simulink subsystem "Joystick_Input_To_Swerve_Drive_sub"  (R2023b)
settings: Solver=VariableStepAuto  StartTime=0.0  StopTime=10.0  RelTol=1e-3
undefined symbols (not defined in the file): Boost_Trigger_High_Speed, Boost_Trigger_Low_Speed, Steering_Abs_Deadband_Range, Steering_Mod_Drv_in, Steering_Mod_Drv_out, Steering_Mod_Str_Rel_in, Steering_Mod_Str_Rel_out, Steering_Relative_Gain
libraries: hdlsllib x5, simulink x4, simulink_extras x1, Controls_Components_lib x1
settings Model: Creator=ander  LastModifiedBy=FIRSTMentor

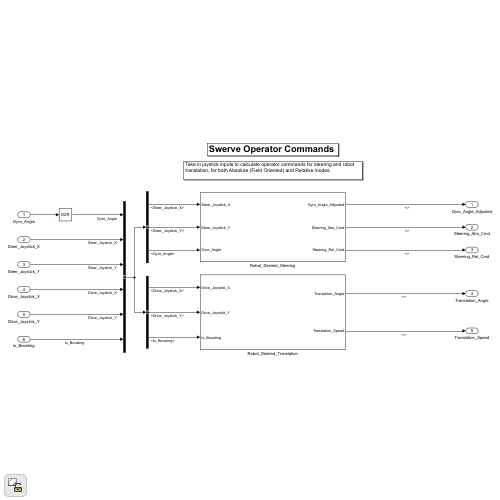
[thumbnail: Simulink's stored preview of the top-level diagram]
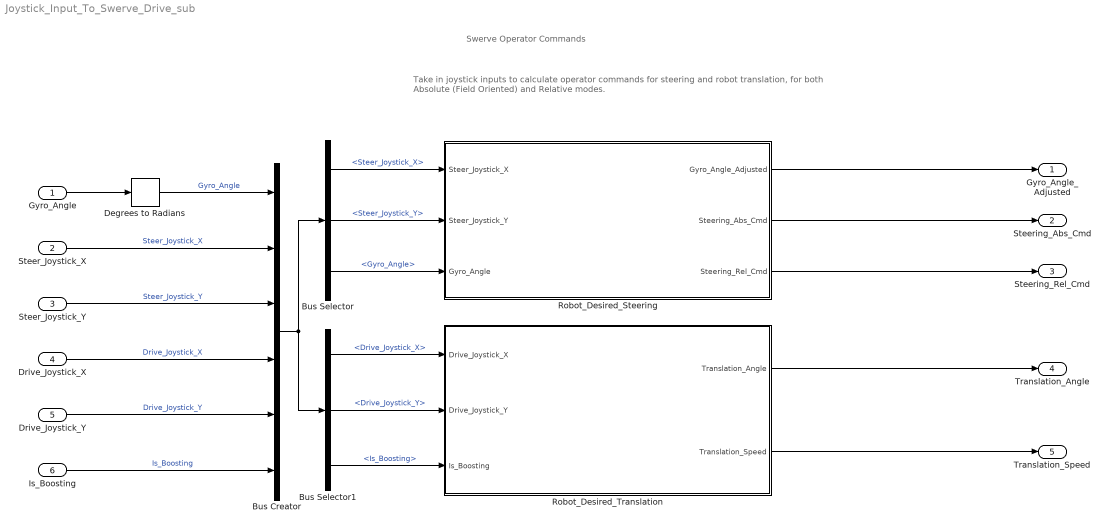
== system Joystick_Input_To_Swerve_Drive_sub ==
  note: Take in joystick inputs to calculate operator commands for steering and robot translation, for both Absolute (Field Oriented) and Relative modes.
  note: Swerve Operator Commands
  Gyro_Angle : Inport
  Steer_Joystick_X : Inport  Port=2
  Steer_Joystick_Y : Inport  Port=3
  Drive_Joystick_X : Inport  Port=4
  Drive_Joystick_Y : Inport  Port=5
  Is_Boosting : Inport  Port=6
  Bus Creator : BusCreator  Inputs=6
  Bus Selector : BusSelector  OutputSignals=Steer_Joystick_X,Steer_Joystick_Y,Gyro_Angle
  Bus Selector1 : BusSelector  OutputSignals=Drive_Joystick_X,Drive_Joystick_Y,Is_Boosting
  Degrees to Radians : simulink_extras/Transformations/Degrees to Radians
  Robot_Desired_Steering : Subsystem
  Robot_Desired_Translation : Subsystem
  Gyro_Angle_Adjusted : Outport
  Steering_Abs_Cmd : Outport  Port=2
  Steering_Rel_Cmd : Outport  Port=3
  Translation_Angle : Outport  Port=4
  Translation_Speed : Outport  Port=5
  wires:
  Drive_Joystick_X/1 -> Bus Creator/4  "Drive_Joystick_X"
  Drive_Joystick_Y/1 -> Bus Creator/5  "Drive_Joystick_Y"
  Steer_Joystick_X/1 -> Bus Creator/2  "Steer_Joystick_X"
  Bus Selector1/1 -> Robot_Desired_Translation/1(Drive_Joystick_X)  "<Drive_Joystick_X>"
  Bus Selector1/2 -> Robot_Desired_Translation/2(Drive_Joystick_Y)  "<Drive_Joystick_Y>"
  Steer_Joystick_Y/1 -> Bus Creator/3  "Steer_Joystick_Y"
  Degrees to Radians/1 -> Bus Creator/1  "Gyro_Angle"
  Gyro_Angle/1 -> Degrees to Radians/1
  Bus Creator/1 -> Bus Selector/1, Bus Selector1/1
  Robot_Desired_Translation/2(Translation_Speed) -> Translation_Speed/1
  Robot_Desired_Translation/1(Translation_Angle) -> Translation_Angle/1
  Bus Selector/1 -> Robot_Desired_Steering/1(Steer_Joystick_X)  "<Steer_Joystick_X>"
  Bus Selector/2 -> Robot_Desired_Steering/2(Steer_Joystick_Y)  "<Steer_Joystick_Y>"
  Bus Selector/3 -> Robot_Desired_Steering/3(Gyro_Angle)  "<Gyro_Angle>"
  Robot_Desired_Steering/1(Gyro_Angle_Adjusted) -> Gyro_Angle_Adjusted/1
  Robot_Desired_Steering/2(Steering_Abs_Cmd) -> Steering_Abs_Cmd/1
  Robot_Desired_Steering/3(Steering_Rel_Cmd) -> Steering_Rel_Cmd/1
  Is_Boosting/1 -> Bus Creator/6  "Is_Boosting"
  Bus Selector1/3 -> Robot_Desired_Translation/3(Is_Boosting)  "<Is_Boosting>"

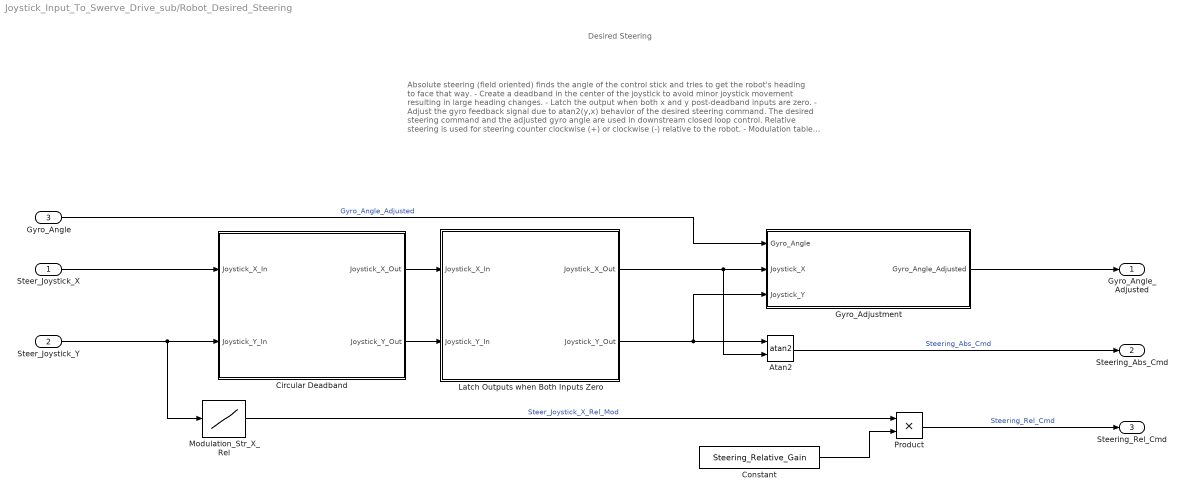
== system Joystick_Input_To_Swerve_Drive_sub/Robot_Desired_Steering ==
  note: Absolute steering (field oriented) finds the angle of the control stick and tries to get the robot's heading to face that way.
      | - Create a deadband in the center of the joystick to avoid minor joystick movement resulting in large heading changes.
      | - Latch the output when both x and y post-deadband inputs are zero.
      | - Adjust the gyro feedback signal due to atan2(y,x) behavior of the desired steering command. The desired steering command and the adjusted gyro angle are used in downstream closed loop control.
      |
      | Relative steering is used for steering counter clockwise (+) or clockwise (-) relative to the robot.
      | - Modulation table for joystick input. Only one axis of the steering joystck is used.
      | - The gain block adjusts how fast the robot will rotate.
  note: Desired Steering
  Steer_Joystick_X : Inport
  Steer_Joystick_Y : Inport  Port=2
  Gyro_Angle : Inport  Port=3
  Atan2 : Trigonometry  Operator=atan2
  Circular Deadband : Subsystem
  Constant : Constant  Value=Steering_Relative_Gain
  Gyro_Adjustment : Subsystem
  Latch Outputs when Both Inputs Zero : Subsystem
  Modulation_Str_X_Rel : Lookup_n-D  NumberOfTableDimensions=1  BreakpointsForDimension1=Steering_Mod_Str_Rel_in  Table=Steering_Mod_Str_Rel_out  ExtrapMethod=Clip  InternalRulePriority=Speed  RndMeth=Simplest
  Product : Product
  Gyro_Angle_Adjusted : Outport
  Steering_Abs_Cmd : Outport  Port=2
  Steering_Rel_Cmd : Outport  Port=3
  wires:
  Latch Outputs when Both Inputs Zero/1(Joystick_X_Out) -> Gyro_Adjustment/2(Joystick_X), Atan2/2
  Circular Deadband/1(Joystick_X_Out) -> Latch Outputs when Both Inputs Zero/1(Joystick_X_In)
  Circular Deadband/2(Joystick_Y_Out) -> Latch Outputs when Both Inputs Zero/2(Joystick_Y_In)
  Steer_Joystick_Y/1 -> Circular Deadband/2(Joystick_Y_In), Modulation_Str_X_Rel/1
  Latch Outputs when Both Inputs Zero/2(Joystick_Y_Out) -> Atan2/1, Gyro_Adjustment/3(Joystick_Y)
  Gyro_Adjustment/1(Gyro_Angle_Adjusted) -> Gyro_Angle_Adjusted/1
  Gyro_Angle/1 -> Gyro_Adjustment/1(Gyro_Angle)  "Gyro_Angle_Adjusted"
  Atan2/1 -> Steering_Abs_Cmd/1  "Steering_Abs_Cmd"
  Constant/1 -> Product/2
  Product/1 -> Steering_Rel_Cmd/1  "Steering_Rel_Cmd"
  Steer_Joystick_X/1 -> Circular Deadband/1(Joystick_X_In)
  Modulation_Str_X_Rel/1 -> Product/1  "Steer_Joystick_X_Rel_Mod"

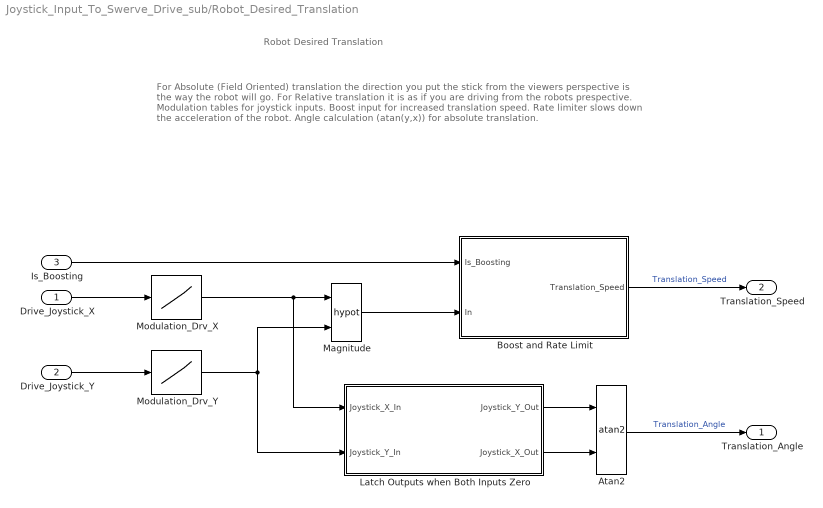
== system Joystick_Input_To_Swerve_Drive_sub/Robot_Desired_Translation ==
  note: Robot Desired Translation
  note: For Absolute (Field Oriented) translation the direction you put the stick from the viewers perspective is the way the robot will go.
      |
      | For Relative translation it is as if you are driving from the robots prespective.
      |
      | Modulation tables for joystick inputs.
      | Boost input for increased translation speed.
      | Rate limiter slows down the acceleration of the robot.
      | Angle calculation (atan(y,x)) for absolute translation.
  Drive_Joystick_X : Inport
  Drive_Joystick_Y : Inport  Port=2
  Is_Boosting : Inport  Port=3
  Atan2 : Trigonometry  Operator=atan2
  Boost and Rate Limit : Subsystem
  Latch Outputs when Both Inputs Zero : Subsystem
  Magnitude : Math  Operator=hypot
  Modulation_Drv_X : Lookup_n-D  NumberOfTableDimensions=1  BreakpointsForDimension1=Steering_Mod_Drv_in  Table=Steering_Mod_Drv_out  ExtrapMethod=Clip  InternalRulePriority=Speed  RndMeth=Simplest
  Modulation_Drv_Y : Lookup_n-D  NumberOfTableDimensions=1  BreakpointsForDimension1=Steering_Mod_Drv_in  Table=Steering_Mod_Drv_out  ExtrapMethod=Clip  InternalRulePriority=Speed  RndMeth=Simplest
  Translation_Angle : Outport
  Translation_Speed : Outport  Port=2
  wires:
  Modulation_Drv_Y/1 -> Magnitude/2, Latch Outputs when Both Inputs Zero/2(Joystick_Y_In)
  Latch Outputs when Both Inputs Zero/1(Joystick_Y_Out) -> Atan2/1
  Latch Outputs when Both Inputs Zero/2(Joystick_X_Out) -> Atan2/2
  Is_Boosting/1 -> Boost and Rate Limit/1(Is_Boosting)
  Boost and Rate Limit/1(Translation_Speed) -> Translation_Speed/1  "Translation_Speed"
  Modulation_Drv_X/1 -> Magnitude/1, Latch Outputs when Both Inputs Zero/1(Joystick_X_In)
  Atan2/1 -> Translation_Angle/1  "Translation_Angle"
  Magnitude/1 -> Boost and Rate Limit/2(In)
  Drive_Joystick_X/1 -> Modulation_Drv_X/1
  Drive_Joystick_Y/1 -> Modulation_Drv_Y/1

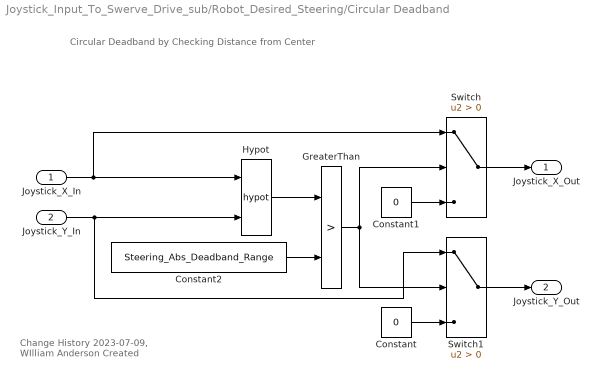
== system Joystick_Input_To_Swerve_Drive_sub/Robot_Desired_Steering/Circular Deadband ==
  note: Circular Deadband by Checking Distance from Center
  note: Change History
      | 2023-07-09, WIlliam Anderson
      | Created
  Joystick_X_In : Inport
  Joystick_Y_In : Inport  Port=2
  Constant : Constant  Value=0
  Constant1 : Constant  Value=0
  Constant2 : Constant  Value=Steering_Abs_Deadband_Range
  GreaterThan : RelationalOperator  Operator=>  OutDataTypeStr=boolean  RndMeth=Simplest  InputSameDT=off
  Hypot : Math  Operator=hypot
  Switch : Switch  Criteria=u2 > Threshold  SaturateOnIntegerOverflow=off  InputSameDT=off
  Switch1 : Switch  Criteria=u2 > Threshold  SaturateOnIntegerOverflow=off  InputSameDT=off
  Joystick_X_Out : Outport
  Joystick_Y_Out : Outport  Port=2
  wires:
  GreaterThan/1 -> Switch1/2, Switch/2
  Constant2/1 -> GreaterThan/2
  Hypot/1 -> GreaterThan/1
  Joystick_Y_In/1 -> Hypot/2, Switch1/1
  Joystick_X_In/1 -> Switch/1, Hypot/1
  Constant1/1 -> Switch/3
  Constant/1 -> Switch1/3
  Switch/1 -> Joystick_X_Out/1
  Switch1/1 -> Joystick_Y_Out/1

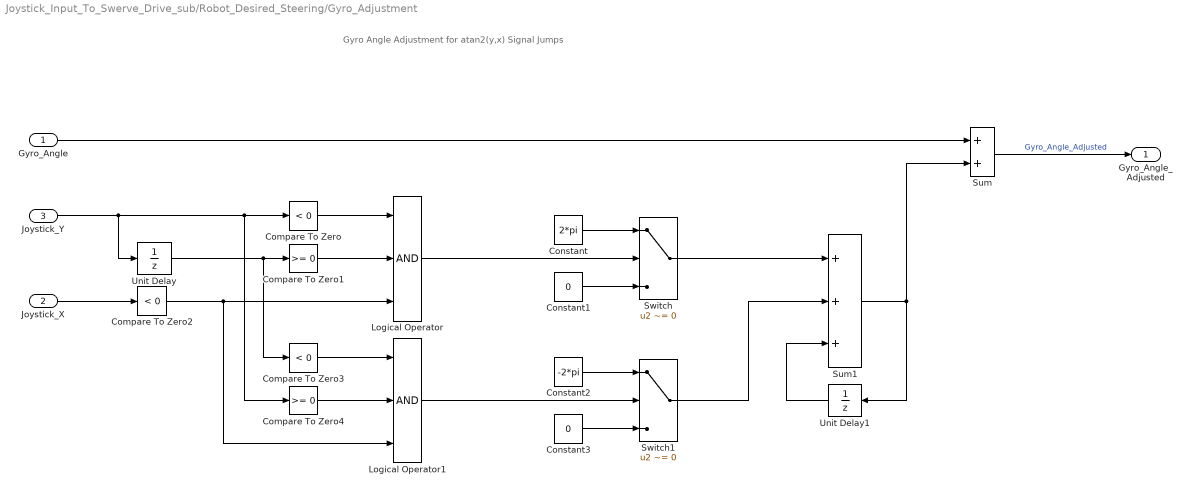
== system Joystick_Input_To_Swerve_Drive_sub/Robot_Desired_Steering/Gyro_Adjustment ==
  note: Gyro Angle Adjustment for atan2(y,x) Signal Jumps
  Gyro_Angle : Inport
  Joystick_X : Inport  Port=2
  Joystick_Y : Inport  Port=3
  Compare To Zero : hdlsllib/Logic and Bit Operations/Compare To Zero  relop=<  OutDataTypeStr=boolean
  Compare To Zero1 : hdlsllib/Logic and Bit Operations/Compare To Zero  relop=>=  OutDataTypeStr=boolean
  Compare To Zero2 : hdlsllib/Logic and Bit Operations/Compare To Zero  relop=<  OutDataTypeStr=boolean
  Compare To Zero3 : hdlsllib/Logic and Bit Operations/Compare To Zero  relop=<  OutDataTypeStr=boolean
  Compare To Zero4 : hdlsllib/Logic and Bit Operations/Compare To Zero  relop=>=  OutDataTypeStr=boolean
  Constant : Constant  Value=2*pi
  Constant1 : Constant  Value=0
  Constant2 : Constant  Value=-2*pi
  Constant3 : Constant  Value=0
  Logical Operator : Logic  Inputs=3  AllPortsSameDT=off  OutDataTypeStr=boolean
  Logical Operator1 : Logic  Inputs=3  AllPortsSameDT=off  OutDataTypeStr=boolean
  Sum : Sum  Inputs=2
  Sum1 : Sum  Inputs=3
  Switch : Switch  Criteria=u2 ~= 0  SaturateOnIntegerOverflow=off  InputSameDT=off
  Switch1 : Switch  Criteria=u2 ~= 0  SaturateOnIntegerOverflow=off  InputSameDT=off
  Unit Delay : UnitDelay  SampleTime=-1  HasFrameUpgradeWarning=on
  Unit Delay1 : UnitDelay  SampleTime=-1  HasFrameUpgradeWarning=on
  Gyro_Angle_Adjusted : Outport
  wires:
  Joystick_Y/1 -> Compare To Zero4/1, Compare To Zero/1, Unit Delay/1
  Unit Delay/1 -> Compare To Zero3/1, Compare To Zero1/1
  Compare To Zero/1 -> Logical Operator/1
  Compare To Zero1/1 -> Logical Operator/2
  Constant/1 -> Switch/1
  Constant1/1 -> Switch/3
  Logical Operator/1 -> Switch/2
  Gyro_Angle/1 -> Sum/1
  Sum/1 -> Gyro_Angle_Adjusted/1  "Gyro_Angle_Adjusted"
  Sum1/1 -> Sum/2, Unit Delay1/1
  Switch/1 -> Sum1/1
  Unit Delay1/1 -> Sum1/3
  Joystick_X/1 -> Compare To Zero2/1
  Compare To Zero2/1 -> Logical Operator1/3, Logical Operator/3
  Compare To Zero3/1 -> Logical Operator1/1
  Compare To Zero4/1 -> Logical Operator1/2
  Logical Operator1/1 -> Switch1/2
  Constant3/1 -> Switch1/3
  Constant2/1 -> Switch1/1
  Switch1/1 -> Sum1/2

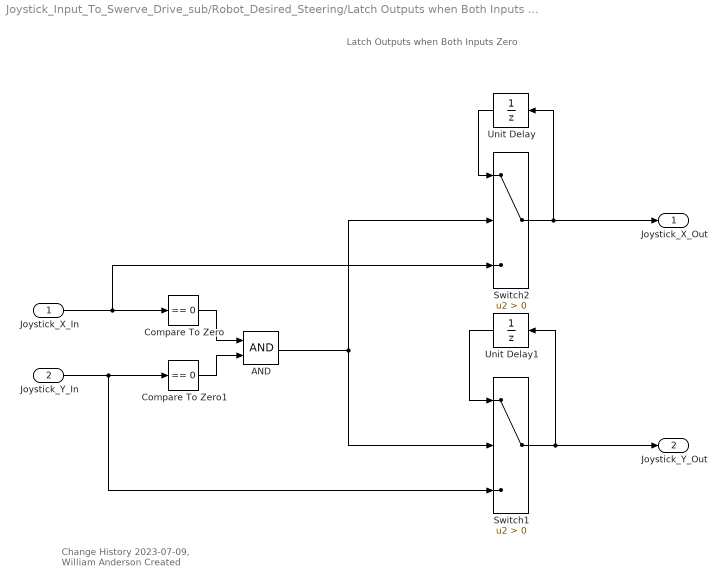
== system Joystick_Input_To_Swerve_Drive_sub/Robot_Desired_Steering/Latch Outputs when Both Inputs Zero ==
  note: Latch Outputs when Both Inputs Zero
  note: Change History
      | 2023-07-09, William Anderson
      | Created
  Joystick_X_In : Inport
  Joystick_Y_In : Inport  Port=2
  AND : Logic  AllPortsSameDT=off  OutDataTypeStr=boolean
  Compare To Zero : simulink/Logic and Bit Operations/Compare To Zero  relop===  OutDataTypeStr=boolean
  Compare To Zero1 : simulink/Logic and Bit Operations/Compare To Zero  relop===  OutDataTypeStr=boolean
  Switch1 : Switch  Criteria=u2 > Threshold  SaturateOnIntegerOverflow=off  InputSameDT=off
  Switch2 : Switch  Criteria=u2 > Threshold  SaturateOnIntegerOverflow=off  InputSameDT=off
  Unit Delay : UnitDelay  SampleTime=-1  HasFrameUpgradeWarning=on
  Unit Delay1 : UnitDelay  SampleTime=-1  HasFrameUpgradeWarning=on
  Joystick_X_Out : Outport
  Joystick_Y_Out : Outport  Port=2
  wires:
  Unit Delay1/1 -> Switch1/1
  Unit Delay/1 -> Switch2/1
  AND/1 -> Switch2/2, Switch1/2
  Compare To Zero/1 -> AND/1
  Compare To Zero1/1 -> AND/2
  Joystick_Y_In/1 -> Compare To Zero1/1, Switch1/3
  Joystick_X_In/1 -> Compare To Zero/1, Switch2/3
  Switch2/1 -> Unit Delay/1, Joystick_X_Out/1
  Switch1/1 -> Unit Delay1/1, Joystick_Y_Out/1

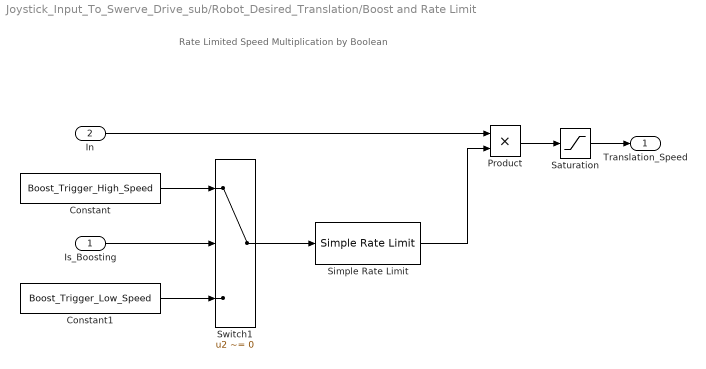
== system Joystick_Input_To_Swerve_Drive_sub/Robot_Desired_Translation/Boost and Rate Limit ==
  note: Rate Limited Speed Multiplication by Boolean
  Is_Boosting : Inport
  In : Inport  Port=2
  Constant : Constant  Value=Boost_Trigger_High_Speed
  Constant1 : Constant  Value=Boost_Trigger_Low_Speed
  Product : Product
  Saturation : Saturate  UpperLimit=Boost_Trigger_High_Speed  LowerLimit=-Boost_Trigger_High_Speed
  Simple Rate Limit : Controls_Components_lib/Simple Rate Limit  Rate_Limit_Inc=Boost_Trigger_Increasing_Limit  Rate_Limit_Dec=Boost_Trigger_Decreasing_Limit
  Switch1 : Switch  Criteria=u2 ~= 0  SaturateOnIntegerOverflow=off  InputSameDT=off
  Translation_Speed : Outport
  wires:
  Saturation/1 -> Translation_Speed/1
  Simple Rate Limit/1 -> Product/2
  Product/1 -> Saturation/1
  In/1 -> Product/1
  Switch1/1 -> Simple Rate Limit/1
  Constant1/1 -> Switch1/3
  Constant/1 -> Switch1/1
  Is_Boosting/1 -> Switch1/2

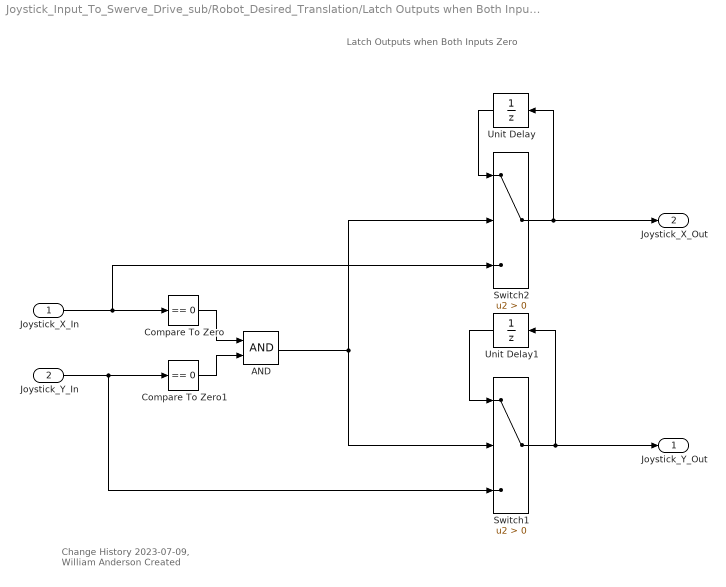
== system Joystick_Input_To_Swerve_Drive_sub/Robot_Desired_Translation/Latch Outputs when Both Inputs Zero ==
  note: Latch Outputs when Both Inputs Zero
  note: Change History
      | 2023-07-09, William Anderson
      | Created
  Joystick_X_In : Inport
  Joystick_Y_In : Inport  Port=2
  AND : Logic  AllPortsSameDT=off  OutDataTypeStr=boolean
  Compare To Zero : simulink/Logic and Bit Operations/Compare To Zero  relop===  OutDataTypeStr=boolean
  Compare To Zero1 : simulink/Logic and Bit Operations/Compare To Zero  relop===  OutDataTypeStr=boolean
  Switch1 : Switch  Criteria=u2 > Threshold  SaturateOnIntegerOverflow=off  InputSameDT=off
  Switch2 : Switch  Criteria=u2 > Threshold  SaturateOnIntegerOverflow=off  InputSameDT=off
  Unit Delay : UnitDelay  SampleTime=-1  HasFrameUpgradeWarning=on
  Unit Delay1 : UnitDelay  SampleTime=-1  HasFrameUpgradeWarning=on
  Joystick_Y_Out : Outport
  Joystick_X_Out : Outport  Port=2
  wires:
  Unit Delay1/1 -> Switch1/1
  Unit Delay/1 -> Switch2/1
  AND/1 -> Switch2/2, Switch1/2
  Compare To Zero/1 -> AND/1
  Compare To Zero1/1 -> AND/2
  Joystick_Y_In/1 -> Compare To Zero1/1, Switch1/3
  Joystick_X_In/1 -> Compare To Zero/1, Switch2/3
  Switch2/1 -> Unit Delay/1, Joystick_X_Out/1
  Switch1/1 -> Unit Delay1/1, Joystick_Y_Out/1
